simulink model "CONTROL_COMPARATION"  (R2023a)
settings: Solver=VariableStepAuto  StartTime=0.0  StopTime=6  RelTol=1e-3
values from neighbouring files (symbols this model uses):
  A = E1*F    [CONTROL_ROLL_OVER.m]    (also in Modelo_roll_control.m; State_space_robust.m; calc_KMax1.m; calc_KMax2.m)
  B = E1*G    [CONTROL_ROLL_OVER.m]    (also in Modelo_roll_control.m; State_space_robust.m; calc_KMax1.m; calc_KMax2.m)
  C = eye(4)    [CONTROL_ROLL_OVER.m]    (also in Modelo_roll_control.m; State_space_robust.m)
  D = zeros(4,1)    [CONTROL_ROLL_OVER.m]    (also in Modelo_roll_control.m = zeros(1,4); State_space_robust.m = zeros(1,4))
  k_h2 = H_2_gain(A,B,B2,C2,D22)    [CONTROL_ROLL_OVER.m]    (also in Modelo_roll_control.m; State_space_robust.m)
  k_inf = H_inf(A,B,B2,C1,D12,D11)    [CONTROL_ROLL_OVER.m]    (also in Modelo_roll_control.m; State_space_robust.m)
  k_l1 = L_1(A,B,B2,C3,D32,D31,lambda)    [CONTROL_ROLL_OVER.m]    (also in Modelo_roll_control.m; State_space_robust.m)
  k_LQ = LQ(Cz,Dzu,A,B,0)    [CONTROL_ROLL_OVER.m]    (also in LQ.m = double(Y)*inv(double(P)); Modelo_roll_control.m; State_space_robust.m)
  kH2Hinf = H_2_H_inf(A,B,B2,C2,D22,C1,D12,D11,a,b)    [CONTROL_ROLL_OVER.m]    (also in Modelo_roll_control.m; State_space_robust.m)
  W = B    [CONTROL_ROLL_OVER.m]    (also in Modelo_roll_control.m; State_space_robust.m; calc_KMax1.m; calc_KMax2.m)
undefined symbols (not defined in the file or in its folder): sigbuilder_block
settings Model: Creator=csanc  LastModifiedBy=csanc

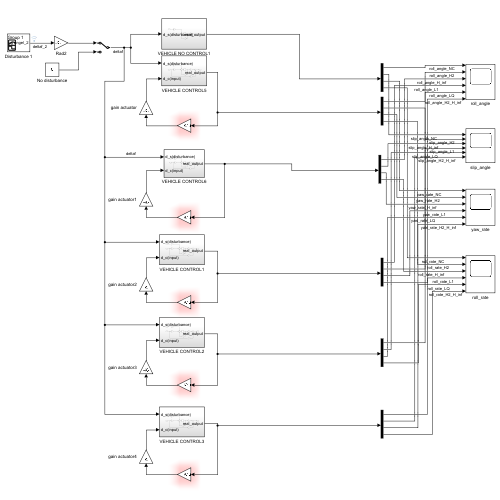
[thumbnail: Simulink's stored preview of the top-level diagram]
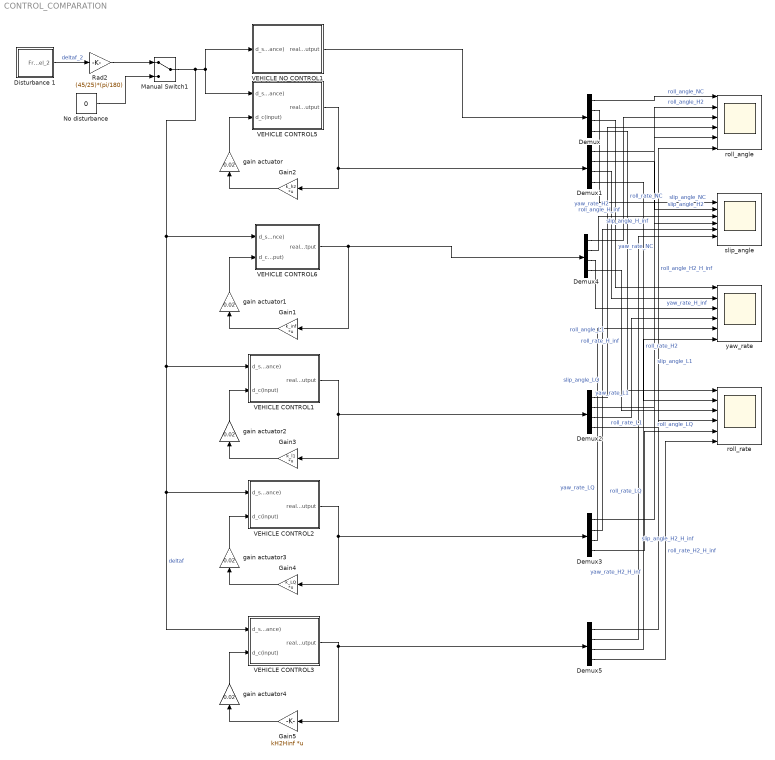
== system CONTROL_COMPARATION ==
  Demux{,1..5} (6 alike) : Demux
  Disturbance 1 : Subsystem  Tag=STV Subsys  LoadFcn=sigbuilder_block('load');  StartFcn=sigbuilder_block('start');  StopFcn=sigbuilder_block('stop');  ClipboardFcn=sigbuilder_block('clipboard');  mask(Sigbuilder block){tuvar=[0:10]}
      mask help: Simulink:masks:SigbuilderBlock_MD
      mask init:
      | if ~strcmp(get_param(bdroot(gcbh),'SimulationStatus'),'stopped') tuvar = sigbuilder_block('maskInit'); end
      settings: CopyFcn=sigbuilder_block('copy');  DeleteFcn=sigbuilder_block('delete');  ModelCloseFcn=sigbuilder_block('modelClose');  PreSaveFcn=sigbuilder_block('preSave');  PauseFcn=sigbuilder_block('pause');  ContinueFcn=sigbuilder_block('continue');  NameChangeFcn=sigbuilder_block('namechange');  OpenFcn=sigbuilder_block('open',[265.8 141.6 550.8 400.2 ]);  CloseFcn=sigbuilder_block('close');
      mask Display: plot(0, 0, 100, 100,[2, 2, 32, 32, 2], [68, 8, 8, 68, 68],[32, 2], [38, 38], [32, 19, 2],[53, 60, 44], [32, 17, 17, 2],[16, 16, 31, 31]);txt = getActiveGroup(gcbh);text(2, 100, txt,'verticalAlignment', 'top');
  Gain1 : Gain  Gain=k_inf  Multiplication=Matrix(K*u)
  Gain2 : Gain  Gain=k_h2  Multiplication=Matrix(K*u)
  Gain3 : Gain  Gain=k_l1  Multiplication=Matrix(K*u)
  Gain4 : Gain  Gain=k_LQ  Multiplication=Matrix(K*u)
  Gain5 : Gain  Gain=kH2Hinf  Multiplication=Matrix(K*u)
  Manual Switch1 : ManualSwitch
  No disturbance : Constant  Value=0
  Rad2 : Gain  Gain=(45/25)*(pi/180)
  VEHICLE CONTROL1 : Subsystem
  VEHICLE CONTROL2 : Subsystem
  VEHICLE CONTROL3 : Subsystem
  VEHICLE CONTROL5 : Subsystem
  VEHICLE CONTROL6 : Subsystem
  VEHICLE NO CONTROL1 : Subsystem
  gain actuator{,1..4} (5 alike) : Gain  Gain=0.02
  roll_angle : Scope  NumInputPorts=6
  roll_rate : Scope  NumInputPorts=6
  slip_angle : Scope  NumInputPorts=6
  yaw_rate : Scope  NumInputPorts=6
  wires:
  Gain2/1 -> gain actuator/1
  Rad2/1 -> Manual Switch1/1
  VEHICLE CONTROL5/1(real_output) -> Demux1/1, Gain2/1
  No disturbance/1 -> Manual Switch1/2
  gain actuator/1 -> VEHICLE CONTROL5/2(d_c(input))
  Disturbance 1/1(Front steering angel_2) -> Rad2/1  "deltaf_2"
  Gain1/1 -> gain actuator1/1
  Manual Switch1/1 -> VEHICLE CONTROL6/1(d_s(disturbance)), VEHICLE CONTROL1/1(d_s(disturbance)), VEHICLE CONTROL3/1(d_s(disturbance)), VEHICLE CONTROL2/1(d_s(disturbance)), VEHICLE NO CONTROL1/1(d_s(disturbance)), VEHICLE CONTROL5/1(d_s(disturbance))  "deltaf"
  Gain3/1 -> gain actuator2/1
  VEHICLE CONTROL1/1(real_output) -> Demux2/1, Gain3/1
  Gain4/1 -> gain actuator3/1
  VEHICLE CONTROL2/1(real_output) -> Demux3/1, Gain4/1
  Gain5/1 -> gain actuator4/1
  VEHICLE CONTROL3/1(real_output) -> Gain5/1, Demux5/1
  VEHICLE NO CONTROL1/1(real_output) -> Demux/1
  Demux/1 -> roll_angle/1  "roll_angle_NC"
  Demux1/1 -> roll_angle/2  "roll_angle_H2"
  Demux4/1 -> roll_angle/3  "roll_angle_H_inf"
  Demux2/1 -> roll_angle/4  "roll_angle_L1"
  Demux3/1 -> roll_angle/5  "roll_angle_LQ"
  Demux5/1 -> roll_angle/6  "roll_angle_H2_H_inf"
  Demux/2 -> slip_angle/1  "slip_angle_NC"
  Demux1/2 -> slip_angle/2  "slip_angle_H2"
  Demux4/2 -> slip_angle/3  "slip_angle_H_inf"
  Demux2/2 -> slip_angle/4  "slip_angle_L1"
  Demux3/2 -> slip_angle/5  "slip_angle_LQ"
  Demux5/2 -> slip_angle/6  "slip_angle_H2_H_inf"
  Demux/3 -> yaw_rate/1  "yaw_rate_NC"
  Demux1/3 -> yaw_rate/2  "yaw_rate_H2"
  Demux4/3 -> yaw_rate/3  "yaw_rate_H_inf"
  Demux2/3 -> yaw_rate/4  "yaw_rate_L1"
  Demux3/3 -> yaw_rate/5  "yaw_rate_LQ"
  Demux5/3 -> yaw_rate/6  "yaw_rate_H2_H_inf"
  Demux/4 -> roll_rate/1  "roll_rate_NC"
  Demux1/4 -> roll_rate/2  "roll_rate_H2"
  Demux4/4 -> roll_rate/3  "roll_rate_H_inf"
  Demux2/4 -> roll_rate/4  "roll_rate_L1"
  Demux3/4 -> roll_rate/5  "roll_rate_LQ"
  Demux5/4 -> roll_rate/6  "roll_rate_H2_H_inf"
  gain actuator1/1 -> VEHICLE CONTROL6/2(d_c(input))
  VEHICLE CONTROL6/1(real_output) -> Gain1/1, Demux4/1
  gain actuator2/1 -> VEHICLE CONTROL1/2(d_c(input))
  gain actuator3/1 -> VEHICLE CONTROL2/2(d_c(input))
  gain actuator4/1 -> VEHICLE CONTROL3/2(d_c(input))

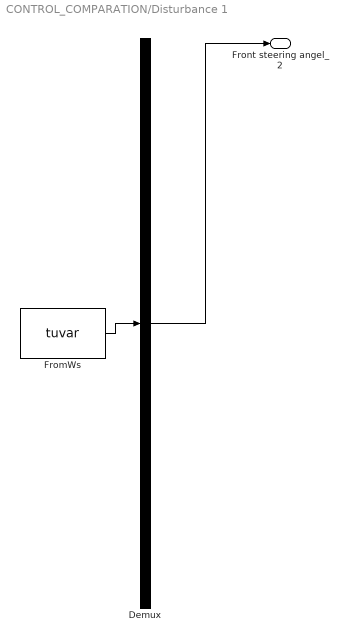
== system CONTROL_COMPARATION/Disturbance 1 ==
  Demux : Demux  Tag=STV Demux  Outputs=1
      settings: DisplayOption=none
  FromWs : FromWorkspace  Tag=STV FromWs  VariableName=tuvar
      SigBuilderData=|
      | common.afterFinalStr = 'Extrapolate'
      | common.sampleTime = 0
      | dataSet.timeRange = [0 3]
      | dataSet.name = 'Group 1'
      | sbobj.Groups.Name = 'Group 1'
      | sbobj.Groups.Signals.Name = 'Front steering angel_2'
      | sbobj.Groups.Signals.XData = [0 0.187490625469 0.374981250937 0.562471876406 0.749962501875 0.937453127344 1.12494375281 1.31243437828 1.49992500375 1.68741562922 1.87490625469 2.06239688016 2.24988750562 2.43737813109 2.62486875656 2.81235938203 2.9998500075 3]
      | sbobj.Groups.Signals.YData = [0 0.565685424949 0.8 0.565685424949 9.79717439318e-17 -0.565685424949 -0.8 -0.565685424949 0 0 0 0 0 0 0 0 0 0]
      | sbobj.Groups.TimeRange = [0 3]
  Front steering angel_2 : Outport  Tag=STV Outport
  wires:
  FromWs/1 -> Demux/1
  Demux/1 -> Front steering angel_2/1

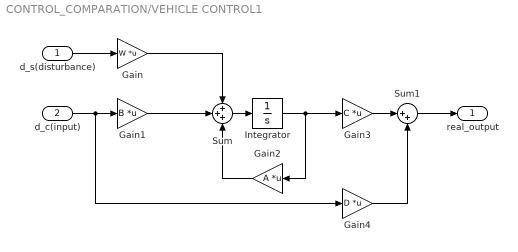
== system CONTROL_COMPARATION/VEHICLE CONTROL1 ==
  d_s(disturbance) : Inport
  d_c(input) : Inport  Port=2
  Gain : Gain  Gain=W  Multiplication=Matrix(K*u)
  Gain1 : Gain  Gain=B  Multiplication=Matrix(K*u)
  Gain2 : Gain  Gain=A  Multiplication=Matrix(K*u)
  Gain3 : Gain  Gain=C  Multiplication=Matrix(K*u)
  Gain4 : Gain  Gain=D  Multiplication=Matrix(K*u)
  Integrator : Integrator  InitialCondition=[0, 0, 0, 0]
  Sum : Sum  Inputs=+++
  Sum1 : Sum  Inputs=|++
  real_output : Outport
  wires:
  Gain1/1 -> Sum/2
  Gain4/1 -> Sum1/2
  d_s(disturbance)/1 -> Gain/1
  Integrator/1 -> Gain3/1, Gain2/1
  Gain/1 -> Sum/1
  Sum1/1 -> real_output/1
  Gain3/1 -> Sum1/1
  Sum/1 -> Integrator/1
  Gain2/1 -> Sum/3
  d_c(input)/1 -> Gain4/1, Gain1/1

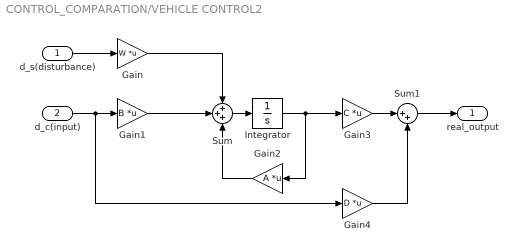
== system CONTROL_COMPARATION/VEHICLE CONTROL2 ==
  d_s(disturbance) : Inport
  d_c(input) : Inport  Port=2
  Gain : Gain  Gain=W  Multiplication=Matrix(K*u)
  Gain1 : Gain  Gain=B  Multiplication=Matrix(K*u)
  Gain2 : Gain  Gain=A  Multiplication=Matrix(K*u)
  Gain3 : Gain  Gain=C  Multiplication=Matrix(K*u)
  Gain4 : Gain  Gain=D  Multiplication=Matrix(K*u)
  Integrator : Integrator  InitialCondition=[0, 0, 0, 0]
  Sum : Sum  Inputs=+++
  Sum1 : Sum  Inputs=|++
  real_output : Outport
  wires:
  Gain1/1 -> Sum/2
  Gain4/1 -> Sum1/2
  d_s(disturbance)/1 -> Gain/1
  Integrator/1 -> Gain3/1, Gain2/1
  Gain/1 -> Sum/1
  Sum1/1 -> real_output/1
  Gain3/1 -> Sum1/1
  Sum/1 -> Integrator/1
  Gain2/1 -> Sum/3
  d_c(input)/1 -> Gain4/1, Gain1/1

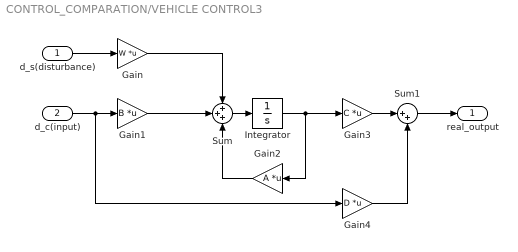
== system CONTROL_COMPARATION/VEHICLE CONTROL3 ==
  d_s(disturbance) : Inport
  d_c(input) : Inport  Port=2
  Gain : Gain  Gain=W  Multiplication=Matrix(K*u)
  Gain1 : Gain  Gain=B  Multiplication=Matrix(K*u)
  Gain2 : Gain  Gain=A  Multiplication=Matrix(K*u)
  Gain3 : Gain  Gain=C  Multiplication=Matrix(K*u)
  Gain4 : Gain  Gain=D  Multiplication=Matrix(K*u)
  Integrator : Integrator  InitialCondition=[0, 0, 0, 0]
  Sum : Sum  Inputs=+++
  Sum1 : Sum  Inputs=|++
  real_output : Outport
  wires:
  Gain1/1 -> Sum/2
  Gain4/1 -> Sum1/2
  d_s(disturbance)/1 -> Gain/1
  Integrator/1 -> Gain3/1, Gain2/1
  Gain/1 -> Sum/1
  Sum1/1 -> real_output/1
  Gain3/1 -> Sum1/1
  Sum/1 -> Integrator/1
  Gain2/1 -> Sum/3
  d_c(input)/1 -> Gain4/1, Gain1/1

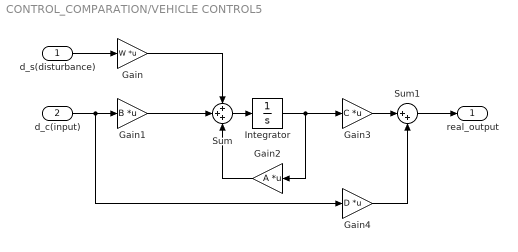
== system CONTROL_COMPARATION/VEHICLE CONTROL5 ==
  d_s(disturbance) : Inport
  d_c(input) : Inport  Port=2
  Gain : Gain  Gain=W  Multiplication=Matrix(K*u)
  Gain1 : Gain  Gain=B  Multiplication=Matrix(K*u)
  Gain2 : Gain  Gain=A  Multiplication=Matrix(K*u)
  Gain3 : Gain  Gain=C  Multiplication=Matrix(K*u)
  Gain4 : Gain  Gain=D  Multiplication=Matrix(K*u)
  Integrator : Integrator  InitialCondition=[0, 0, 0, 0]
  Sum : Sum  Inputs=+++
  Sum1 : Sum  Inputs=|++
  real_output : Outport
  wires:
  Gain1/1 -> Sum/2
  Gain4/1 -> Sum1/2
  d_s(disturbance)/1 -> Gain/1
  Integrator/1 -> Gain3/1, Gain2/1
  Gain/1 -> Sum/1
  Sum1/1 -> real_output/1
  Gain3/1 -> Sum1/1
  Sum/1 -> Integrator/1
  Gain2/1 -> Sum/3
  d_c(input)/1 -> Gain4/1, Gain1/1

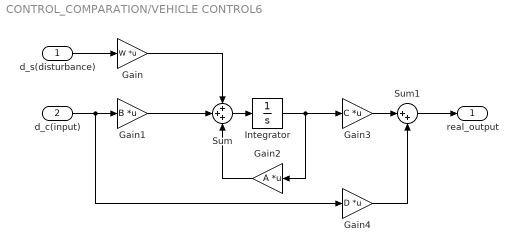
== system CONTROL_COMPARATION/VEHICLE CONTROL6 ==
  d_s(disturbance) : Inport
  d_c(input) : Inport  Port=2
  Gain : Gain  Gain=W  Multiplication=Matrix(K*u)
  Gain1 : Gain  Gain=B  Multiplication=Matrix(K*u)
  Gain2 : Gain  Gain=A  Multiplication=Matrix(K*u)
  Gain3 : Gain  Gain=C  Multiplication=Matrix(K*u)
  Gain4 : Gain  Gain=D  Multiplication=Matrix(K*u)
  Integrator : Integrator  InitialCondition=[0, 0, 0, 0]
  Sum : Sum  Inputs=+++
  Sum1 : Sum  Inputs=|++
  real_output : Outport
  wires:
  Gain1/1 -> Sum/2
  Gain4/1 -> Sum1/2
  d_s(disturbance)/1 -> Gain/1
  Integrator/1 -> Gain3/1, Gain2/1
  Gain/1 -> Sum/1
  Sum1/1 -> real_output/1
  Gain3/1 -> Sum1/1
  Sum/1 -> Integrator/1
  Gain2/1 -> Sum/3
  d_c(input)/1 -> Gain4/1, Gain1/1

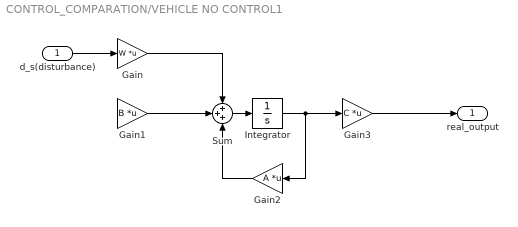
== system CONTROL_COMPARATION/VEHICLE NO CONTROL1 ==
  d_s(disturbance) : Inport
  Gain : Gain  Gain=W  Multiplication=Matrix(K*u)
  Gain1 : Gain  Gain=B  Multiplication=Matrix(K*u)
  Gain2 : Gain  Gain=A  Multiplication=Matrix(K*u)
  Gain3 : Gain  Gain=C  Multiplication=Matrix(K*u)
  Integrator : Integrator  InitialCondition=[0, 0, 0, 0]
  Sum : Sum  Inputs=+++
  real_output : Outport
  wires:
  Gain1/1 -> Sum/2
  d_s(disturbance)/1 -> Gain/1
  Integrator/1 -> Gain3/1, Gain2/1
  Gain/1 -> Sum/1
  Gain3/1 -> real_output/1
  Sum/1 -> Integrator/1
  Gain2/1 -> Sum/3
